simulink model "ResouceAllocation"  (R2026a)
settings: Solver=VariableStepAuto  StopTime=20.0

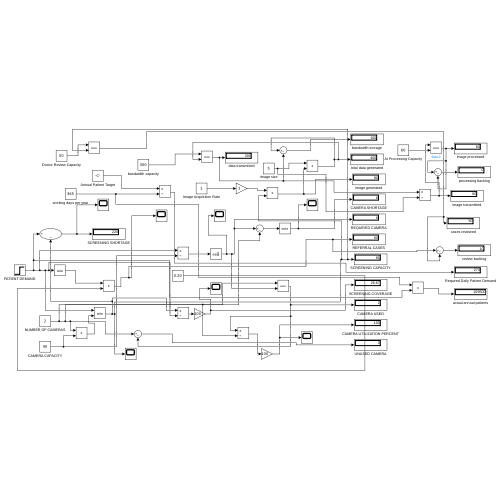
[thumbnail: Simulink's stored preview of the top-level diagram]
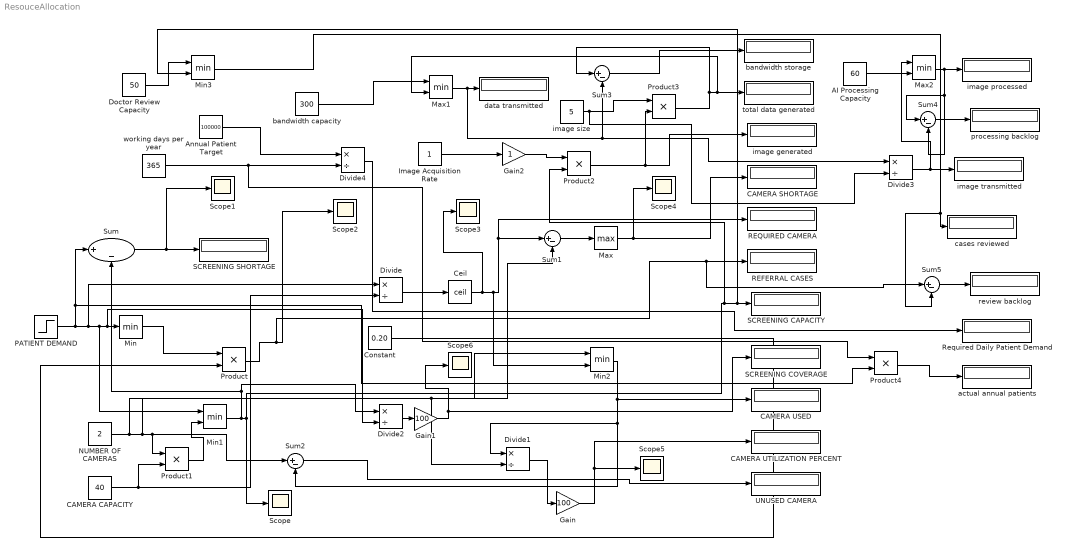
== system ResouceAllocation ==
  AI Processing Capacity : Constant  Value=60
  Annual Patient Target : Constant  Value=100000
  CAMERA CAPACITY : Constant  Value=40
  CAMERA SHORTAGE : Display
  CAMERA USED : Display
  CAMERA UTILIZATION PERCENT : Display
  Ceil : Rounding  Operator=ceil
  Constant : Constant  Value=0.20
  Divide{,1..4} (5 alike) : Product  Inputs=*/
  Doctor Review Capacity : Constant  Value=50
  Gain : Gain  Gain=100
  Gain1 : Gain  Gain=100
  Gain2 : Gain
  Image Acquisition Rate : Constant
  Max : MinMax  Function=max
  Max1 : MinMax  Inputs=2
  Max2 : MinMax  Inputs=2
  Min : MinMax
  Min1 : MinMax  Inputs=2
  Min2 : MinMax  Inputs=2
  Min3 : MinMax  Inputs=2
  NUMBER OF CAMERAS : Constant  Value=2
  PATIENT DEMAND : Step  Time=10  InitialValue=100  FinalValue=300  SampleTime=0
  Product{,1..4} (5 alike) : Product
  REFERRAL CASES : Display
  REQUIRED CAMERA : Display
  Required Daily Patient Demand : Display
  SCREENING CAPACITY : Display
  SCREENING COVERAGE : Display
  SCREENING SHORTAGE : Display
  Scope{,1..6} (7 alike) : Scope
      Scope settings: ActiveDisplayYMinimum=14.40910628577182  ActiveDisplayYMaximum=93.569197762172081
      Scope1 settings: ActiveDisplayYMinimum=-81.081561233003612  ActiveDisplayYMaximum=104.73009369483711
      Scope2 settings: ActiveDisplayYMinimum=-15.977162673711206  ActiveDisplayYMaximum=38.391692541208059  DataLoggingVariableName=ScopeData2
      Scope3 settings: ActiveDisplayYMinimum=1.75  ActiveDisplayYMaximum=4.25  DataLoggingVariableName=ScopeData3
      Scope4 settings: ActiveDisplayYMinimum=-0.24999999999999994  ActiveDisplayYMaximum=2.25  DataLoggingVariableName=ScopeData4
      Scope5 settings: ActiveDisplayYMinimum=90  ActiveDisplayYMaximum=110  DataLoggingVariableName=ScopeData5
      Scope6 settings: ActiveDisplayYMinimum=47.5  ActiveDisplayYMaximum=105.83333333333333  DataLoggingVariableName=ScopeData6
  Sum{,1..5} (6 alike) : Sum  Inputs=|+-
  UNUSED CAMERA : Display
  actual annual patients : Display
  bandwidth capacity : Constant  Value=300
  bandwidth storage : Display
  cases reviewed : Display
  data transmitted : Display
  image generated : Display
  image processed : Display
  image size : Constant  Value=5
  image transmitted : Display
  processing backlog : Display
  review backlog : Display
  total data generated : Display
  working days per year : Constant  Value=365
  wires:
  Min/1 -> Product/1
  Constant/1 -> Product/2
  Product/1 -> Scope2/1, Sum5/1, REFERRAL CASES/1
  PATIENT DEMAND/1 -> Product4/2, Sum/1, Divide2/2, Min/1, Min1/1, Divide/1
  Sum/1 -> Scope1/1, SCREENING SHORTAGE/1
  NUMBER OF CAMERAS/1 -> Divide1/2, Sum1/2, Sum2/1, Product1/1, Min2/1
  CAMERA CAPACITY/1 -> Divide/2, Product1/2
  Product1/1 -> Min1/2
  Min1/1 -> Sum/2, Divide2/1, Scope/1, Product2/2, Min3/2, SCREENING CAPACITY/1
  Divide/1 -> Ceil/1
  Ceil/1 -> Scope3/1, Min2/2, Sum1/1, REQUIRED CAMERA/1
  Sum1/1 -> Max/1
  Min2/1 -> Divide1/1, Sum2/2, CAMERA USED/1
  Sum2/1 -> UNUSED CAMERA/1
  Divide1/1 -> Gain/1
  Gain/1 -> Scope5/1, CAMERA UTILIZATION PERCENT/1
  Divide2/1 -> Gain1/1
  Gain1/1 -> Scope6/1, SCREENING COVERAGE/1
  Max/1 -> Scope4/1, CAMERA SHORTAGE/1
  Image Acquisition Rate/1 -> Gain2/1
  Gain2/1 -> Product2/1
  Product2/1 -> Product3/2, image generated/1
  image size/1 -> Divide3/2, Product3/1
  Product3/1 -> Sum3/1, Max1/2, total data generated/1
  bandwidth capacity/1 -> Max1/1
  Max1/1 -> Divide3/1, Sum3/2, data transmitted/1
  Sum3/1 -> bandwidth storage/1
  AI Processing Capacity/1 -> Max2/2
  Max2/1 -> Sum4/1, Sum4/2, image processed/1
  Sum4/1 -> processing backlog/1
  Divide3/1 -> Max2/1, image transmitted/1
  Doctor Review Capacity/1 -> Min3/1
  Min3/1 -> Sum5/2, cases reviewed/1
  Sum5/1 -> review backlog/1
  Annual Patient Target/1 -> Divide4/1
  Divide4/1 -> Required Daily Patient Demand/1
  working days per year/1 -> Product4/1, Divide4/2
  Product4/1 -> actual annual patients/1
